simulink model "soc_range_doppler_top"  (R2023b)
settings: Solver=VariableStepAuto  StartTime=0.0  StopTime=stoptime  RelTol=1e-3  EnableMultiTasking=on
PreLoadFcn:
  | soc_range_doppler_init
InitFcn:
  | hsb.blkcb2.defineTypes
  | soc_range_doppler_init
model workspace (MAT data in the model file):
  mmap = soc.memmap.MemoryMap
  mmap.isMapValid = 1
  mmap.controllerInfo = soc.memmap.MemController
  mmap.controllerInfo.memPSRange = {'2', 'G'}
  mmap.controllerInfo.memPLBaseAddr = '0x500000000'
  mmap.controllerInfo.memPLRange = {'4', 'G'}
  mmap.controllerInfo.memPLBaseAddrMMU = {9, '0'}
  mmap.controllerInfo.regBaseAddr = '0xA0000000'
  mmap.controllerInfo.regAddrRange = {'256', 'M'}
  mmap.map(1) = soc.memmap.MapParams
  mmap.map(1).type = 'PS Memory Region'
  mmap.map(1).name = 'AXI4-Stream to Software'
  mmap.map(1).baseAddr = '0x00000000'
  mmap.map(1).range = {'4096', 'K'}
  mmap.map(1).path = 'soc_range_doppler_top/AXI4-Stream to Software'
  mmap.map(2) = soc.memmap.MapParams
  mmap.map(2).type = 'User Component'
  mmap.map(2).name = 'Radar Target Emulator'
  mmap.map(2).baseAddr = '0xA0000000'
  mmap.map(2).range = {'64', 'K'}
  mmap.map(2).path = 'soc_range_doppler_fpga/Radar Target Emulator'
  mmap.map(2).regs(1) = soc.memmap.IPCoreRegParams
  mmap.map(2).regs(1).register = 'HDL Coder registers'
  mmap.map(2).regs(1).offset = '0x0000 - 0x00FF'
  mmap.map(2).regs(1).vectorlength = 'N/A'
  mmap.map(2).regs(1).type = 'Reserved'
  mmap.map(2).regs(1).reserved = 1
  mmap.map(2).regs(2) = soc.memmap.IPCoreRegParams
  mmap.map(2).regs(2).blkname = 'Radar Target Emulator'
  mmap.map(2).regs(2).register = 'Target_Emulator_Doppler_Inc'
  mmap.map(2).regs(2).offset = '0x0100'
  mmap.map(2).regs(2).vectorlength = '4'
  mmap.map(2).regs(2).type = 'Processor write channel'
  mmap.map(2).regs(3) = soc.memmap.IPCoreRegParams
  mmap.map(2).regs(3).blkname = 'Radar Target Emulator'
  mmap.map(2).regs(3).register = 'Target_Emulator_Range_Delay'
  mmap.map(2).regs(3).offset = '0x0120'
  mmap.map(2).regs(3).vectorlength = '4'
  mmap.map(2).regs(3).type = 'Processor write channel'
  mmap.map(2).regs(4) = soc.memmap.IPCoreRegParams
  mmap.map(2).regs(4).blkname = 'Radar Target Emulator'
  mmap.map(2).regs(4).register = 'Target_Emulator_Gain'
  mmap.map(2).regs(4).offset = '0x0140'
  mmap.map(2).regs(4).vectorlength = '4'
  mmap.map(2).regs(4).type = 'Processor write channel'
  mmap.map(2).regs(5) = soc.memmap.IPCoreRegParams
  mmap.map(2).regs(5).blkname = 'Radar Target Emulator'
  mmap.map(2).regs(5).register = 'Target_Emulator_Channel_Enable'
  mmap.map(2).regs(5).offset = '0x0160'
  mmap.map(2).regs(5).vectorlength = '4'
  mmap.map(2).regs(5).type = 'Processor write channel'
  mmap.map(3) = soc.memmap.MapParams
  mmap.map(3).type = 'User Component'
  mmap.map(3).name = 'Range Doppler Tx-Rx'
  mmap.map(3).baseAddr = '0xA0010000'
  mmap.map(3).range = {'64', 'K'}
  mmap.map(3).path = 'soc_range_doppler_fpga/Range Doppler Tx-Rx'
  mmap.map(3).regs(1) = soc.memmap.IPCoreRegParams
  mmap.map(3).regs(1).register = 'HDL Coder registers'
  mmap.map(3).regs(1).offset = '0x0000 - 0x00FF'
  mmap.map(3).regs(1).vectorlength = 'N/A'
  mmap.map(3).regs(1).type = 'Reserved'
  mmap.map(3).regs(1).reserved = 1
  mmap.map(3).regs(2) = soc.memmap.IPCoreRegParams
  mmap.map(3).regs(2).blkname = 'Range Doppler Tx-Rx'
  mmap.map(3).regs(2).register = 'Tx_Gain'
  mmap.map(3).regs(2).offset = '0x0100'
  mmap.map(3).regs(2).vectorlength = '1'
  mmap.map(3).regs(2).type = 'Processor write channel'
  mmap.map(3).regs(3) = soc.memmap.IPCoreRegParams
  mmap.map(3).regs(3).blkname = 'Range Doppler Tx-Rx'
  mmap.map(3).regs(3).register = 'CPI_Start'
  mmap.map(3).regs(3).offset = '0x0104'
  mmap.map(3).regs(3).vectorlength = '1'
  mmap.map(3).regs(3).type = 'Processor write channel'
  mmap.map(3).regs(4) = soc.memmap.IPCoreRegParams
  mmap.map(3).regs(4).blkname = 'Range Doppler Tx-Rx'
  mmap.map(3).regs(4).register = 'CPI_Length'
  mmap.map(3).regs(4).offset = '0x0108'
  mmap.map(3).regs(4).vectorlength = '1'
  mmap.map(3).regs(4).type = 'Processor write channel'
  mmap.map(3).regs(5) = soc.memmap.IPCoreRegParams
  mmap.map(3).regs(5).blkname = 'Range Doppler Tx-Rx'
  mmap.map(3).regs(5).register = 'Rx_Delay_Cycles'
  mmap.map(3).regs(5).offset = '0x010C'
  mmap.map(3).regs(5).vectorlength = '1'
  mmap.map(3).regs(5).type = 'Processor write channel'
  mmap.map(4) = soc.memmap.MapParams
  mmap.map(4).type = 'Implicit Component'
  mmap.map(4).name = 'AXI4-Stream to Software DMA S2MM'
  mmap.map(4).baseAddr = '0xA0020000'
  mmap.map(4).range = {'64', 'K'}
  mmap.map(5) = soc.memmap.MapParams
  mmap.map(5).type = 'Implicit Component'
  mmap.map(5).name = 'RFDataConverter/s_axi'
  mmap.map(5).baseAddr = '0xA3C00000'
  mmap.map(5).range = {'256', 'K'}
  mwTaskManagerKernelLatency = 0
  socicb{1}.Registry = containers.Map
  socicb{1}.Registry.serialization.keys = {34131.0015869}
  socicb{1}.Registry.serialization.values = {1}
  socicb{1}.Registry.serialization.uniformity = 0
  socicb{1}.Registry.serialization.keyType = 'double'
  socicb{1}.Registry.serialization.valueType = 'any'
  socicb{1}.Index = 2
  socicb{2}.Registry = containers.Map
  socicb{2}.Registry.serialization.keys = {}
  socicb{2}.Registry.serialization.values = {}
  socicb{2}.Registry.serialization.uniformity = 0
  socicb{2}.Registry.serialization.keyType = 'double'
  socicb{2}.Registry.serialization.valueType = 'any'
  socicb{2}.Index = 1
  socvcb = containers.Map
  socvcb.serialization.keys = {514.000488281}
  socvcb.serialization.values : function handle (value not decoded)
  socvcb.serialization.uniformity = 0
  socvcb.serialization.keyType = 'double'
  socvcb.serialization.valueType = 'any'
values from neighbouring files (symbols this model uses):
  ConverterSampleRate = 2e9    (= 2000000000)    [soc_range_doppler_init.m]
  FPGAClkRate = Fs/SamplesPerClockCycle    (= 125000000)    [soc_range_doppler_init.m]
  Fs = ConverterSampleRate/DecimInterpFactor    (= 250000000)    [soc_range_doppler_init.m]
  LoopbackDelayCycles = 63    [soc_range_doppler_init.m]
  RxDelayCycles = RngGateSamples/SamplesPerClockCycle + LoopbackDelayCycles*2    [soc_range_doppler_init.m]
  SamplesPerClockCycle = 2    [soc_range_doppler_init.m]
  TsFPGA = 1/FPGAClkRate    (= 8e-09)    [soc_range_doppler_init.m]
  TsHost = 5e-5    (= 5e-05)    [soc_range_doppler_init.m]
  udp_cmd = struct()    [soc_range_doppler_init.m]
undefined symbols (not defined in the file or in its folder): CPILength, D1, D2, I, m, n, P, Q, RngMaxIdx, VelMaxIdx
libraries: prociodatalib x2, dspsrcs4 x2, socmemlib x1, proctasklib x1, xilinxrfsoclib x1
settings Model: ModifiedByFormat=The MathWorks, Inc.  Creator=The MathWorks, Inc.  LastModifiedBy=The MathWorks, Inc.
settings SolverCC: ConcurrentTasks=on  AlgebraicLoopSolver=TrustRegion  PositivePriorityOrder=on  MaxZcPerStep=1
settings DataIOCC: ReturnWorkspaceOutputs=off
settings OptimizationCC: EnhancedBackFolding=on  PassReuseOutputArgsAs=Individual arguments  ZeroExternalMemoryAtStartup=off  ZeroInternalMemoryAtStartup=off  MaxStackSize=64  OptimizeBlockOrder=speed  DifferentSizesBufferReuse=on  OptimizationCustomize=off  EfficientTunableParamExpr=on
settings DebuggingCC: ParameterTunabilityLossMsg=error  UnconnectedInputMsg=warning  UnconnectedOutputMsg=warning  UnconnectedLineMsg=warning
settings HardwareCC: ProdBitPerLong=64  ProdLargestAtomicInteger=LongLong  ProdLargestAtomicFloat=Double  ProdLongLongMode=on  ProdHWDeviceType=ARM Compatible->ARM 64-bit (LP64)  HardwareBoardFeatureSet=SoCBlockset
settings ModelReferenceCC: EnableRefExpFcnMdlSchedulingChecks=on  ModelReferenceNumInstancesAllowed=Single
settings SFSimCC: MATLABDynamicMemAlloc=off
settings RTWCC: Description=Embedded Coder  SystemTargetFile=ert.tlc  HardwareBoard=Xilinx Zynq UltraScale+ RFSoC ZCU111 Evaluation Kit  TLCOptions="-aInlineSetEventsForThisBaseRateFcn=TLC_FALSE -aSuppressMultiTaskScheduler=TLC_FALSE  -aRateBasedStepFcn=0"  TemplateMakefile=ert_default_tmf  Toolchain=Linaro AArch64 Linux v6.3.1  DLArmComputeVersion=19.05
settings CodeAppCC: ForceParamTrailComments=on  IgnoreCustomStorageClasses=off  OperatorAnnotations=on  SimulinkDataObjDesc=on  SFDataObjDesc=on  InsertBlockDesc=on

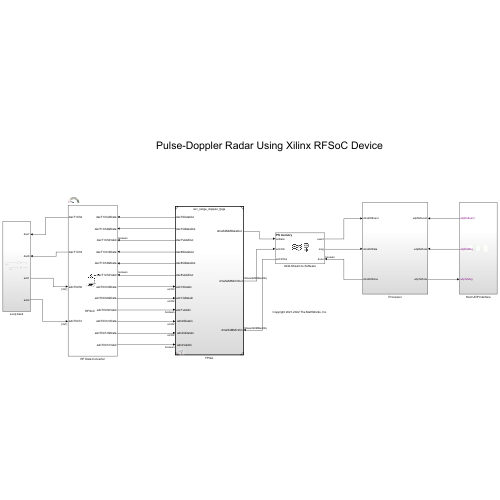
[thumbnail: Simulink's stored preview of the top-level diagram]
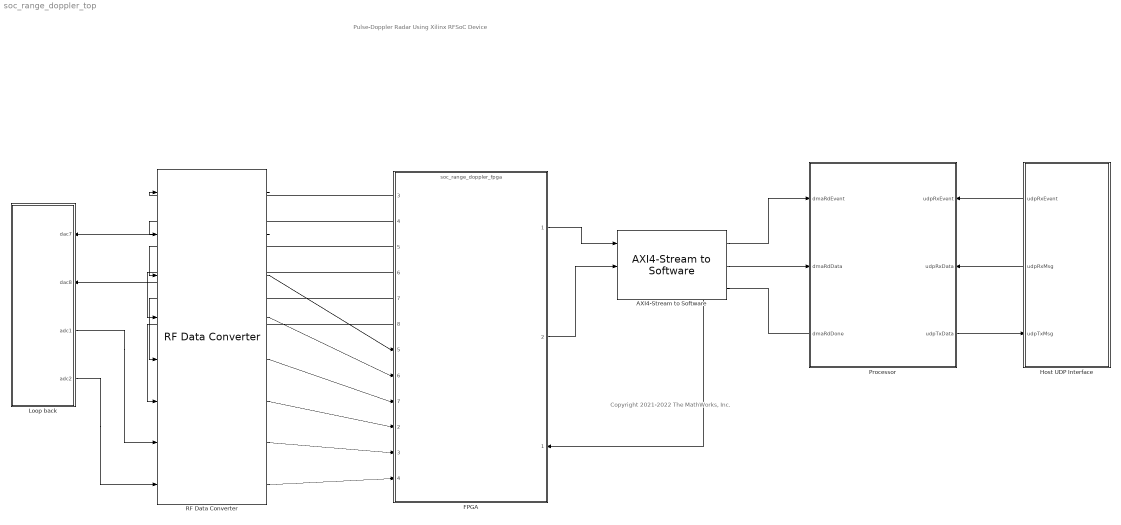
== system soc_range_doppler_top ==
  note: Pulse-Doppler Radar Using Xilinx RFSoC Device
  note: Copyright 2021-2022 The MathWorks, Inc.
  AXI4-Stream to Software : socmemlib/AXI4-Stream to Software  MemorySimulation=Burst accurate  MemorySelection=PS memory  MRNumBuffers=S2MM_DMANumBuffers  BurstLengthWriterChIf=256  FIFODepthWriter=8  FIFOAFullDepthWriter=6  ICClockFrequencyWriter=300  ICDataWidthWriter=64  ChDimensionsWriterChIf=1  ChTypeWriterChIf=uint64  ChFrameSampleTimeWriterChIf=1/FPGAClkRate  ChBitPackedWriterChIf=off  ChDimensionsReaderChIf=S2MM_DMAFrameLength  ChTypeReaderChIf=uint64  LastTargetBoard=Xilinx Zynq UltraScale+ RFSoC ZCU111 Evaluation Kit  MRRegionSize=4194304  MRBufferSize=262144  DiagnosticLevel=No debug
  FPGA : ModelReference  ModelNameDialog=soc_range_doppler_fpga.slx  SimulationMode=Normal  ModelReferenceVersion=1.0
      settings: PortSchema="{\"entries\":[{\"content\":{\"sides\":[{\"content\":{\"connectorIds\":[\"Out3\",\"Out4\",\"Out5\",\"Out6\",\"Out7\",\"Out8\",\"In5\",\"In6\",\"In7\",\"In2\",\"In3\",\"In4\"]},\"type\":\"ConnectorPlacement.EquallySpacedRectSide\",\"uuid\":\"422e8f89-866f-4e63-8b25-cadbd336be37\"},{\"content\":{\"connectorIds\":[\"Out1\",\"Out2\",\"In1\"],\"side\":\"RIGHT\"},\"type\":\"ConnectorPlacement.EquallySpacedRectSide\",\"uuid\":\"dce0ed7e-9928-416e-b2ed-d7d34b81a84a\"},{\"content\":{\"connectorIds\":[],\"side\":\"TOP\"},\"type\":\"ConnectorPlacement.EquallySpacedRectSide\",\"uuid\":\"a6e1b56d-9a0e-41ff-8dbe-5200ba64d569\"}]},\"type\":\"ConnectorPlacement.EquallySpacedConnector\",\"uuid\":\"a650c01e-33da-4d6b-a752-c4fd08663ce5\"}],\"packageUris\":[\"http://schema.mathworks.com/mf0/Connector/R2020b\"],\"version\":\"1.0\"}"
  Host UDP Interface : Subsystem
      settings: PortSchema="{\"entries\":[{\"content\":{\"sides\":[{\"content\":{\"connectorIds\":[\"Out1\",\"Out2\",\"In1\"]},\"type\":\"ConnectorPlacement.EquallySpacedRectSide\",\"uuid\":\"9c3f3ca2-7255-442d-89df-713aeb26e21e\"},{\"content\":{\"connectorIds\":[],\"side\":\"RIGHT\"},\"type\":\"ConnectorPlacement.EquallySpacedRectSide\",\"uuid\":\"e07d2c4c-30b4-495f-acff-78102ba2fb53\"},{\"content\":{\"connectorIds\":[],\"side\":\"TOP\"},\"type\":\"ConnectorPlacement.EquallySpacedRectSide\",\"uuid\":\"853d940a-d21c-462a-929f-98a301461923\"},{\"content\":{\"connectorIds\":[],\"side\":\"HIDDEN\"},\"type\":\"ConnectorPlacement.EquallySpacedRectSide\",\"uuid\":\"ea8c92dd-7626-4add-bd8f-a9d4935d66f8\"}]},\"type\":\"ConnectorPlacement.EquallySpacedConnector\",\"uuid\":\"2455c085-c623-453a-9196-168aa3e9b36f\"}],\"packageUris\":[\"http://schema.mathworks.com/mf0/Connector/R2020b\"],\"version\":\"1.0\"}"
  Loop back : Subsystem
      settings: PortSchema="{\"entries\":[{\"content\":{\"sides\":[{\"content\":{\"connectorIds\":[]},\"type\":\"ConnectorPlacement.EquallySpacedRectSide\",\"uuid\":\"975a5334-a629-4491-b90c-43fa61341479\"},{\"content\":{\"connectorIds\":[\"In1\",\"In2\",\"Out1\",\"Out2\"],\"side\":\"RIGHT\"},\"type\":\"ConnectorPlacement.EquallySpacedRectSide\",\"uuid\":\"05690cce-8672-402a-8253-0f6b9724a041\"},{\"content\":{\"connectorIds\":[],\"side\":\"TOP\"},\"type\":\"ConnectorPlacement.EquallySpacedRectSide\",\"uuid\":\"0d5c0932-fd92-4b6a-b2b9-8137fdfe5c54\"}]},\"type\":\"ConnectorPlacement.EquallySpacedConnector\",\"uuid\":\"05fdaa57-5b6b-4572-a65f-c3b7d5edf9ae\"}],\"packageUris\":[\"http://schema.mathworks.com/mf0/Connector/R2020b\"],\"version\":\"1.0\"}"
  Processor : Subsystem
      settings: PortSchema="{\"entries\":[{\"content\":{\"sides\":[{\"content\":{\"connectorIds\":[\"In1\",\"In2\",\"Out2\"]},\"type\":\"ConnectorPlacement.EquallySpacedRectSide\",\"uuid\":\"fdd8d51e-84cf-4172-ae92-3a2268afb915\"},{\"content\":{\"connectorIds\":[\"In3\",\"In4\",\"Out1\"],\"side\":\"RIGHT\"},\"type\":\"ConnectorPlacement.EquallySpacedRectSide\",\"uuid\":\"e3c7202d-80e2-4cca-8eeb-2f96d776b6b9\"},{\"content\":{\"connectorIds\":[],\"side\":\"TOP\"},\"type\":\"ConnectorPlacement.EquallySpacedRectSide\",\"uuid\":\"d91d78b2-c830-4c1a-8566-0c5cca5f25a7\"}]},\"type\":\"ConnectorPlacement.EquallySpacedConnector\",\"uuid\":\"41410483-7731-4907-8551-24eb7e6a32eb\"}],\"packageUris\":[\"http://schema.mathworks.com/mf0/Connector/R2020b\"],\"version\":\"1.0\"}"
  RF Data Converter : xilinxrfsoclib/RF Data Converter  RFDCSim=Pass-through  tabPromptsCB=0  RFInterface=Customize  digitalInterface=I/Q  dac11Enable=off  dac12Enable=off  dac13Enable=off  dac14Enable=off  dac21Enable=off  dac22Enable=off  dac23Enable=on  dac24Enable=on  dac31Enable=off  dac32Enable=off  dac33Enable=off  dac34Enable=off  dac41Enable=off  dac42Enable=off  dac43Enable=off  dac44Enable=off  matchDACParam=on  dacSampleRate=ConverterSampleRate/1e6  interpolationMode=8  dacSamplesPerCycle=2  dacMixerType=Fine  dacMixerMode=I/Q->Real  dacMixerFrequency=Fs/4  dacNCOFrequency=0.5*ones(1,2)  dacNCOPhase=0*ones(1,2)  invertSyncFilter=off  dacTile1SampleRate=1000  dac11InterpolationMode=2  dac11SamplesPerCycle=2  dac11MixerType=Coarse  dac11MixerMode=I/Q->Real  dac11MixerFrequency=Fs/2  dac11NCOFrequency=0  dac11NCOPhase=0  dac11InvertSyncFilter=off  dac12InterpolationMode=2  dac12SamplesPerCycle=2  dac12MixerType=Coarse  dac12MixerMode=I/Q->Real  dac12MixerFrequency=Fs/2  dac12NCOFrequency=0  dac12NCOPhase=0  dac12InvertSyncFilter=off  dac13InterpolationMode=2  dac13SamplesPerCycle=2  dac13MixerType=Coarse  dac13MixerMode=I/Q->Real  dac13MixerFrequency=Fs/2  dac13NCOFrequency=0  dac13NCOPhase=0  dac13InvertSyncFilter=off  dac14InterpolationMode=2  dac14SamplesPerCycle=2  dac14MixerType=Coarse  dac14MixerMode=I/Q->Real  dac14MixerFrequency=Fs/2  dac14NCOFrequency=0  dac14NCOPhase=0  dac14InvertSyncFilter=off  dacTile2SampleRate=1000  dac21InterpolationMode=2  dac21SamplesPerCycle=2  dac21MixerType=Coarse  dac21MixerMode=I/Q->Real  dac21MixerFrequency=Fs/2  dac21NCOFrequency=0  dac21NCOPhase=0  dac21InvertSyncFilter=off  dac22InterpolationMode=2  dac22SamplesPerCycle=2  dac22MixerType=Coarse  dac22MixerMode=I/Q->Real  dac22MixerFrequency=Fs/2  dac22NCOFrequency=0  dac22NCOPhase=0  dac22InvertSyncFilter=off  dac23InterpolationMode=2  dac23SamplesPerCycle=2  dac23MixerType=Coarse  dac23MixerMode=I/Q->Real  dac23MixerFrequency=Fs/2  dac23NCOFrequency=0  dac23NCOPhase=0  dac23InvertSyncFilter=off  dac24InterpolationMode=2  dac24SamplesPerCycle=2  dac24MixerType=Coarse  dac24MixerMode=I/Q->Real  dac24MixerFrequency=Fs/2  dac24NCOFrequency=0  dac24NCOPhase=0  dac24InvertSyncFilter=off  dacTile3SampleRate=1000  dac31InterpolationMode=2  dac31SamplesPerCycle=2  dac31MixerType=Coarse  dac31MixerMode=I/Q->Real  dac31MixerFrequency=Fs/2  dac31NCOFrequency=0  dac31NCOPhase=0  dac31InvertSyncFilter=off  dac32InterpolationMode=2  dac32SamplesPerCycle=2  dac32MixerType=Coarse  dac32MixerMode=I/Q->Real  dac32MixerFrequency=Fs/2  dac32NCOFrequency=0  dac32NCOPhase=0  dac32InvertSyncFilter=off  dac33InterpolationMode=2  dac33SamplesPerCycle=2  dac33MixerType=Coarse  dac33MixerMode=I/Q->Real  dac33MixerFrequency=Fs/2  dac33NCOFrequency=0  dac33NCOPhase=0  dac33InvertSyncFilter=off  dac34InterpolationMode=2  dac34SamplesPerCycle=2  dac34MixerType=Coarse  dac34MixerMode=I/Q->Real  dac34MixerFrequency=Fs/2  dac34NCOFrequency=0  dac34NCOPhase=0  dac34InvertSyncFilter=off  dacTile4SampleRate=1000  dac41InterpolationMode=2  dac41SamplesPerCycle=2  dac41MixerType=Coarse  dac41MixerMode=I/Q->Real  dac41MixerFrequency=Fs/2  dac41NCOFrequency=0  dac41NCOPhase=0  dac41InvertSyncFilter=off  dac42InterpolationMode=2  dac42SamplesPerCycle=2  dac42MixerType=Coarse  dac42MixerMode=I/Q->Real  dac42MixerFrequency=Fs/2  dac42NCOFrequency=0  dac42NCOPhase=0  dac42InvertSyncFilter=off  dac43InterpolationMode=2  dac43SamplesPerCycle=2  dac43MixerType=Coarse  dac43MixerMode=I/Q->Real  dac43MixerFrequency=Fs/2  dac43NCOFrequency=0  dac43NCOPhase=0  dac43InvertSyncFilter=off  dac44InterpolationMode=2  dac44SamplesPerCycle=2  dac44MixerType=Coarse  dac44MixerMode=I/Q->Real  dac44MixerFrequency=Fs/2  dac44NCOFrequency=0  dac44NCOPhase=0  dac44InvertSyncFilter=off  adc11Enable=on  adc12Enable=on  adc13Enable=off  adc14Enable=off  adc21Enable=off  adc22Enable=off  adc23Enable=off  adc24Enable=off  adc31Enable=off  adc32Enable=off  adc33Enable=off  adc34Enable=off  adc41Enable=off  adc42Enable=off  adc43Enable=off  adc44Enable=off  adcOutUnpackedData=off  matchADCParam=on  adcSampleRate=ConverterSampleRate/1e6  decimationMode=8  adcSamplesPerCycle=2  adcMixerType=Fine  adcMixerMode=Real->I/Q  adcMixerFrequency=-Fs/4  adcNCOFrequency=-0.5*ones(1,2)  adcNCOPhase=0*ones(1,2)  adcTile1SampleRate=1000  adc11DecimationMode=2  adc11SamplesPerCycle=2  adc11MixerType=Coarse  adc11MixerMode=Real->I/Q  adc11MixerFrequency=Fs/2  adc11NCOFrequency=0  adc11NCOPhase=0  adc12DecimationMode=2  adc12SamplesPerCycle=2  adc12MixerType=Coarse  adc12MixerMode=Real->I/Q  adc12MixerFrequency=Fs/2  adc12NCOFrequency=0  adc12NCOPhase=0  adc13DecimationMode=2  adc13SamplesPerCycle=2  adc13MixerType=Coarse  adc13MixerMode=Real->I/Q  adc13MixerFrequency=Fs/2  adc13NCOFrequency=0  adc13NCOPhase=0  adc14DecimationMode=2  adc14SamplesPerCycle=2  adc14MixerType=Coarse  adc14MixerMode=Real->I/Q  adc14MixerFrequency=Fs/2  adc14NCOFrequency=0  adc14NCOPhase=0  adcTile2SampleRate=1000  adc21DecimationMode=2  adc21SamplesPerCycle=2  adc21MixerType=Coarse  adc21MixerMode=Real->I/Q  adc21MixerFrequency=Fs/2  adc21NCOFrequency=0  adc21NCOPhase=0  adc22DecimationMode=2  adc22SamplesPerCycle=2  adc22MixerType=Coarse  adc22MixerMode=Real->I/Q  adc22MixerFrequency=Fs/2  adc22NCOFrequency=0  adc22NCOPhase=0  adc23DecimationMode=2  adc23SamplesPerCycle=2  adc23MixerType=Coarse  adc23MixerMode=Real->I/Q  adc23MixerFrequency=Fs/2  adc23NCOFrequency=0  adc23NCOPhase=0  adc24DecimationMode=2  adc24SamplesPerCycle=2  adc24MixerType=Coarse  adc24MixerMode=Real->I/Q  adc24MixerFrequency=Fs/2  adc24NCOFrequency=0  adc24NCOPhase=0  adcTile3SampleRate=1000  adc31DecimationMode=2  adc31SamplesPerCycle=2  adc31MixerType=Coarse  adc31MixerMode=Real->I/Q  adc31MixerFrequency=Fs/2  adc31NCOFrequency=0  adc31NCOPhase=0  adc32DecimationMode=2  adc32SamplesPerCycle=2  adc32MixerType=Coarse  adc32MixerMode=Real->I/Q  adc32MixerFrequency=Fs/2  adc32NCOFrequency=0  adc32NCOPhase=0  adc33DecimationMode=2  adc33SamplesPerCycle=2  adc33MixerType=Coarse  adc33MixerMode=Real->I/Q  adc33MixerFrequency=Fs/2  adc33NCOFrequency=0  adc33NCOPhase=0  adc34DecimationMode=2  adc34SamplesPerCycle=2  adc34MixerType=Coarse  adc34MixerMode=Real->I/Q  adc34MixerFrequency=Fs/2  adc34NCOFrequency=0  adc34NCOPhase=0  adcTile4SampleRate=1000  adc41DecimationMode=2  adc41SamplesPerCycle=2  adc41MixerType=Coarse  adc41MixerMode=Real->I/Q  adc41MixerFrequency=Fs/2  adc41NCOFrequency=0  adc41NCOPhase=0  adc42DecimationMode=2  adc42SamplesPerCycle=2  adc42MixerType=Coarse  adc42MixerMode=Real->I/Q  adc42MixerFrequency=Fs/2  adc42NCOFrequency=0  adc42NCOPhase=0  adc43DecimationMode=2  adc43SamplesPerCycle=2  adc43MixerType=Coarse  adc43MixerMode=Real->I/Q  adc43MixerFrequency=Fs/2  adc43NCOFrequency=0  adc43NCOPhase=0  adc44DecimationMode=2  adc44SamplesPerCycle=2  adc44MixerType=Coarse  adc44MixerMode=Real->I/Q  adc44MixerFrequency=Fs/2  adc44NCOFrequency=0  adc44NCOPhase=0  multiTileSync=off  externalPLL=off  dacRealTimeNCOPortsEnable=off  adcRealTimeNCOPortsEnable=off  adcRealTimePortsEnable=off  adcThresholdMode=Sticky over  adcThreshold1=0  adcDelayCounter=0  adcThreshold2Mode=Sticky over  adcThreshold2=0  adcThreshold2DelayCounter=0  adc11ThresholdMode=Sticky over  adc11Threshold1=0  adc11DelayCounter=0  adc11Threshold2Mode=Sticky over  adc11Threshold2=0  adc11Threshold2DelayCounter=0  adc12ThresholdMode=Sticky over  adc12Threshold1=0  adc12DelayCounter=0  adc12Threshold2Mode=Sticky over  adc12Threshold2=0  adc12Threshold2DelayCounter=0  adc13ThresholdMode=Sticky over  adc13Threshold1=0  adc13DelayCounter=0  adc13Threshold2Mode=Sticky over  adc13Threshold2=0  adc13Threshold2DelayCounter=0  adc14ThresholdMode=Sticky over  adc14Threshold1=0  adc14DelayCounter=0  adc14Threshold2Mode=Sticky over  adc14Threshold2=0  adc14Threshold2DelayCounter=0  adc21ThresholdMode=Sticky over  adc21Threshold1=0  adc21DelayCounter=0  adc21Threshold2Mode=Sticky over  adc21Threshold2=0  adc21Threshold2DelayCounter=0  adc22ThresholdMode=Sticky over  adc22Threshold1=0  adc22DelayCounter=0  adc22Threshold2Mode=Sticky over  adc22Threshold2=0  adc22Threshold2DelayCounter=0  adc23ThresholdMode=Sticky over  adc23Threshold1=0  adc23DelayCounter=0  adc23Threshold2Mode=Sticky over  adc23Threshold2=0  adc23Threshold2DelayCounter=0  adc24ThresholdMode=Sticky over  adc24Threshold1=0  adc24DelayCounter=0  adc24Threshold2Mode=Sticky over  adc24Threshold2=0  adc24Threshold2DelayCounter=0  adc31ThresholdMode=Sticky over  adc31Threshold1=0  adc31DelayCounter=0  adc31Threshold2Mode=Sticky over  adc31Threshold2=0  adc31Threshold2DelayCounter=0  adc32ThresholdMode=Sticky over  adc32Threshold1=0  adc32DelayCounter=0  adc32Threshold2Mode=Sticky over  adc32Threshold2=0  adc32Threshold2DelayCounter=0  adc33ThresholdMode=Sticky over  adc33Threshold1=0  adc33DelayCounter=0  adc33Threshold2Mode=Sticky over  adc33Threshold2=0  adc33Threshold2DelayCounter=0  adc34ThresholdMode=Sticky over  adc34Threshold1=0  adc34DelayCounter=0  adc34Threshold2Mode=Sticky over  adc34Threshold2=0  adc34Threshold2DelayCounter=0  adc41ThresholdMode=Sticky over  adc41Threshold1=0  adc41DelayCounter=0  adc41Threshold2Mode=Sticky over  adc41Threshold2=0  adc41Threshold2DelayCounter=0  adc42ThresholdMode=Sticky over  adc42Threshold1=0  adc42DelayCounter=0  adc42Threshold2Mode=Sticky over  adc42Threshold2=0  adc42Threshold2DelayCounter=0  adc43ThresholdMode=Sticky over  adc43Threshold1=0  adc43DelayCounter=0  adc43Threshold2Mode=Sticky over  adc43Threshold2=0  adc43Threshold2DelayCounter=0  adc44ThresholdMode=Sticky over  adc44Threshold1=0  adc44DelayCounter=0  adc44Threshold2Mode=Sticky over  adc44Threshold2=0  adc44Threshold2DelayCounter=0
  wires:
  Host UDP Interface/1(udpRxEvent) -> Processor/3(udpRxEvent)
  Processor/1(udpTxData) -> Host UDP Interface/1(udpTxMsg)
  AXI4-Stream to Software/1 -> Processor/1(dmaRdEvent)
  AXI4-Stream to Software/2 -> Processor/2(dmaRdData)
  Host UDP Interface/2(udpRxMsg) -> Processor/4(udpRxData)
  Processor/2(dmaRdDone) -> AXI4-Stream to Software/3
  FPGA/1 -> AXI4-Stream to Software/1
  FPGA/2 -> AXI4-Stream to Software/2
  AXI4-Stream to Software/3 -> FPGA/1
  Loop back/1(adc1) -> RF Data Converter/7
  Loop back/2(adc2) -> RF Data Converter/8
  RF Data Converter/2 -> Loop back/2(dac8)
  RF Data Converter/1 -> Loop back/1(dac7)
  FPGA/3 -> RF Data Converter/1
  FPGA/4 -> RF Data Converter/2
  FPGA/5 -> RF Data Converter/3
  FPGA/6 -> RF Data Converter/4
  FPGA/7 -> RF Data Converter/5
  FPGA/8 -> RF Data Converter/6
  RF Data Converter/3 -> FPGA/5
  RF Data Converter/4 -> FPGA/6
  RF Data Converter/5 -> FPGA/7
  RF Data Converter/6 -> FPGA/2
  RF Data Converter/7 -> FPGA/3
  RF Data Converter/8 -> FPGA/4

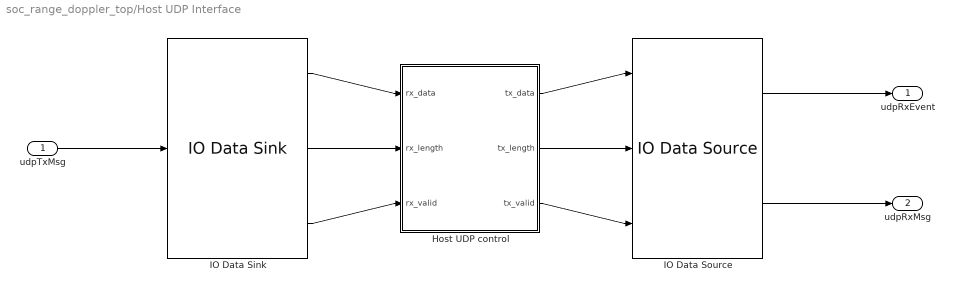
== system soc_range_doppler_top/Host UDP Interface ==
  udpTxMsg : Inport
  Host UDP control : MATLAB Function  TreatAsAtomicUnit=on
  IO Data Sink : prociodatalib/IO Data Sink  OutputSink=To output port  DataTypeStr=single  Dimensions=RngMaxIdx*VelMaxIdx  DeviceType=UDP  EventDataPort=Data  QueueLength=65535  SampleTime=TsHost  EnableDonePort=off
  IO Data Source : prociodatalib/IO Data Source  InputSource=From input port  Value=uint32(1:1024)  ObjectName=[]  DeviceType=UDP  ShowEventPort=off  EventDataPort=Data and Event  QueueLength=1024  DataTypeStr=uint32  Dimensions=1024  ShowDonePort=off  SampleTime=-1  InternalSampleTime=-1
  udpRxEvent : Outport
  udpRxMsg : Outport  Port=2
  wires:
  IO Data Source/2 -> udpRxMsg/1
  IO Data Source/1 -> udpRxEvent/1
  udpTxMsg/1 -> IO Data Sink/1
  IO Data Sink/1 -> Host UDP control/1(rx_data)
  IO Data Sink/2 -> Host UDP control/2(rx_length)
  IO Data Sink/3 -> Host UDP control/3(rx_valid)
  Host UDP control/3(tx_valid) -> IO Data Source/3
  Host UDP control/2(tx_length) -> IO Data Source/2
  Host UDP control/1(tx_data) -> IO Data Source/1

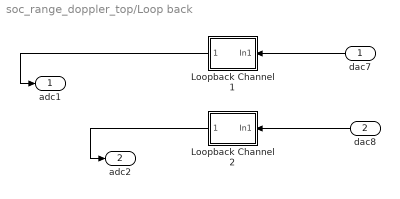
== system soc_range_doppler_top/Loop back ==
  dac7 : Inport
  dac8 : Inport  Port=2
  Loopback Channel 1 : Subsystem
  Loopback Channel 2 : Subsystem
  adc1 : Outport
  adc2 : Outport  Port=2
  wires:
  dac7/1 -> Loopback Channel 1/1(In1)
  Loopback Channel 2/1(Out1) -> adc2/1
  dac8/1 -> Loopback Channel 2/1(In1)
  Loopback Channel 1/1(Out1) -> adc1/1

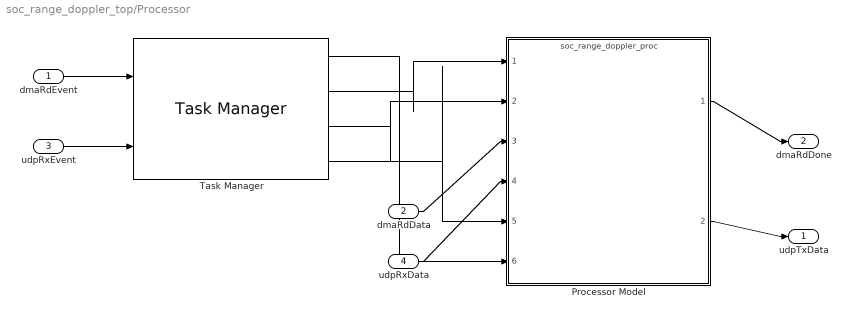
== system soc_range_doppler_top/Processor ==
  dmaRdEvent : Inport
  dmaRdData : Inport  Port=2
  udpRxEvent : Inport  Port=3
  udpRxData : Inport  Port=4
  Processor Model : ModelReference  InputPortMessageModes=n,n,m,m,n,n  OutputPortMessageModes=m,m  ModelNameDialog=soc_range_doppler_proc.slx  SimulationMode=Normal  ScheduleRates=on  CachedPortDiscreteRates=[0.01;0.2]  ModelEventPortInfo=P:D1[0.01][0][0],P:D2[0.2][0][0]  ModelReferenceVersion=1.0
  Task Manager : proctasklib/Task Manager  AllTaskData="[{\"taskName\":\"baseRateTask\",\"taskType\":\"Timer-driven\",\"taskEvent\":\"baseRateTaskEvent\",\"taskPeriod\":\"TsSWBase\",\"taskPriority\":\"51\",\"coreSelection\":\"Specified core\",\"coreNum\":\"0\",\"dropOverranTasks\":false,\"playbackRecorded\":false,\"diagnosticsFile\":\"\",\"taskDurationSource\":\"Dialog\",\"taskDuration\":1E-6,\"taskDurationDeviation\":0,\"logExecutionData\":true,\"logDroppedTasks\":false,\"version\":\"2.6\",\"taskDurationData\":{\"percent\":\"100\",\"mean\":\"1e-06\",\"dev\":\"0\",\"min\":\"1e-06\",\"max\":\"1e-06\"},\"taskEventSource\":\"Internal\",\"taskEventSourceAssignmentType\":\"AutoAssigned\",\"taskEventSourceType\":\"Unspecified\",\"taskEventGroup\":\"Unspecified\",\"taskEventInterrupt\":\"Unspecified\",\"taskEventOrder\":1,\"taskDisablePremption\":false,\"taskClearInterruptFlagsAtEndOfEvent\":false},{\"taskName\":\"dataReadTask\",\"taskType\":\"Event-driven\",\"taskEvent\":\"dataReadTaskEvent\",\"taskPeriod\":\"0.1\",\"taskPriority\":\"50\",\"coreSelection\":\"Specified core\",\"coreNum\":\"1\",\"dropOverranTasks\":false,\"playbackRecorded\":false,\"diagnosticsFile\":\"\",\"taskDurationSource\":\"Dialog\",\"taskDuration\":1E-6,\"taskDurationDeviation\":0,\"logExecutionData\":true,\"logDroppedTasks\":false,\"version\":\"2.6\",\"taskDurationData\":{\"percent\":[\"100\"],\"mean\":[\"10e-6\"],\"dev\":[\"0\"],\"min\":[\"8e-6\"],\"max\":[\"12e-6\"]},\"taskEventSource\":\"AXI4-Stream to Software\",\"taskEventSourceAssignmentType\":\"AutoAssigned\",\"taskEventSourceType\":\"Stream\",\"taskEventGroup\":\"Unspecified\",\"taskEventInterrupt\":\"Unspecified\",\"taskEventOrder\":1,\"taskDisablePremption\":false,\"taskClearInterruptFlagsAtEndOfEvent\":false},{\"taskName\":\"udpRxTask\",\"taskType\":\"Event-driven\",\"taskEvent\":\"udpRxTaskEvent\",\"taskPeriod\":\"0.1\",\"taskPriority\":\"45\",\"coreSelection\":\"Specified core\",\"coreNum\":\"0\",\"dropOverranTasks\":false,\"playbackRecorded\":false,\"diagnosticsFile\":\"\",\"taskDurationSource\":\"Dialog\",\"taskDuration\":1E-6,\"taskDurationDeviation\":0,\"logExecutionData\":true,\"logDroppedTasks\":false,\"version\":\"2.6\",\"taskDurationData\":{\"percent\":[\"100\"],\"mean\":[\"1.55e-6\"],\"dev\":[\"0\"],\"min\":[\"1.5e-6\"],\"max\":[\"1.6e-6\"]},\"taskEventSource\":\"IO Data Source\",\"taskEventSourceAssignmentType\":\"AutoAssigned\",\"taskEventSourceType\":\"\",\"taskEventGroup\":\"Unspecified\",\"taskEventInterrupt\":\"Unspecified\",\"taskEventOrder\":1,\"taskDisablePremption\":false,\"taskClearInterruptFlagsAtEndOfEvent\":false},{\"taskName\":\"radarTargetUpdateTask\",\"taskType\":\"Timer-driven\",\"taskEvent\":\"newTask1Event\",\"taskPeriod\":\"TsTargetUpdate\",\"taskPriority\":\"51\",\"coreSelection\":\"Specified core\",\"coreNum\":\"2\",\"dropOverranTasks\":false,\"playbackRecorded\":false,\"diagnosticsFile\":\"\",\"taskDurationSource\":\"Dialog\",\"taskDuration\":1E-6,\"taskDurationDeviation\":0,\"logExecutionData\":true,\"logDroppedTasks\":false,\"version\":\"2.6\",\"taskDurationData\":{\"percent\":\"100\",\"mean\":\"1e-06\",\"dev\":\"0\",\"min\":\"1e-06\",\"max\":\"1e-06\"},\"taskEventSource\":\"Internal\",\"taskEventSourceAssignmentType\":\"AutoAssigned\",\"taskEventSourceType\":\"Unspecified\",\"taskEventGroup\":\"Unspecified\",\"taskEventInterrupt\":\"Unspecified\",\"taskEventOrder\":1,\"taskDisablePremption\":false,\"taskClearInterruptFlagsAtEndOfEvent\":false}]"  EnableTaskSimulation=on  StreamToSDI=on  WriteToFile=off  OverwriteFile=off  SupportEventPorts=on  UseScheduleEditor=off  CustomizationInfo=''
  udpTxData : Outport
  dmaRdDone : Outport  Port=2
  wires:
  Processor Model/1 -> dmaRdDone/1
  dmaRdData/1 -> Processor Model/3
  udpRxData/1 -> Processor Model/4
  Processor Model/2 -> udpTxData/1
  dmaRdEvent/1 -> Task Manager/1
  udpRxEvent/1 -> Task Manager/2
  Task Manager/2 -> Processor Model/1
  Task Manager/3 -> Processor Model/2
  Task Manager/1 -> Processor Model/6
  Task Manager/4 -> Processor Model/5

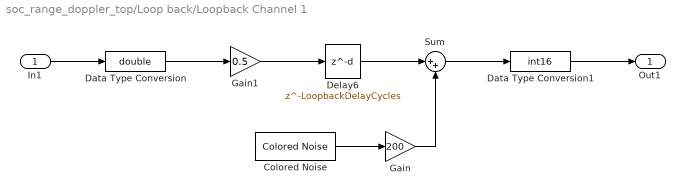
== system soc_range_doppler_top/Loop back/Loopback Channel 1 ==
  In1 : Inport
  Colored Noise : dspsrcs4/Colored Noise  Color=white  InverseFrequencyPower=1  BoundedOutput=off  NumChannels=1  OutputDataType=double  SamplesPerFrame=SamplesPerClockCycle*2  SampleTime=TsFPGA/(SamplesPerClockCycle*2)  RandomStream=mt19937ar with seed  Seed=68  SimulateUsing=Interpreted execution
  Data Type Conversion : DataTypeConversion  OutDataTypeStr=double  SaturateOnIntegerOverflow=off  RndMeth=Floor
  Data Type Conversion1 : DataTypeConversion  OutDataTypeStr=int16  SaturateOnIntegerOverflow=off  RndMeth=Floor
  Delay6 : Delay  DelayLength=LoopbackDelayCycles
  Gain : Gain  Gain=200
  Gain1 : Gain  Gain=0.5
  Sum : Sum  Inputs=|++
  Out1 : Outport
  wires:
  Gain1/1 -> Delay6/1
  In1/1 -> Data Type Conversion/1
  Data Type Conversion/1 -> Gain1/1
  Data Type Conversion1/1 -> Out1/1
  Delay6/1 -> Sum/1
  Colored Noise/1 -> Gain/1
  Gain/1 -> Sum/2
  Sum/1 -> Data Type Conversion1/1

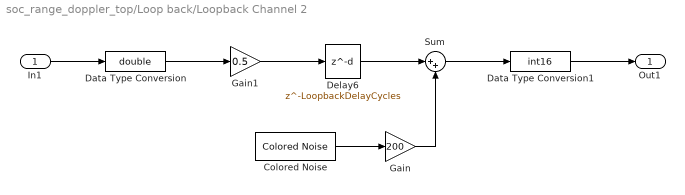
== system soc_range_doppler_top/Loop back/Loopback Channel 2 ==
  In1 : Inport
  Colored Noise : dspsrcs4/Colored Noise  Color=white  InverseFrequencyPower=1  BoundedOutput=off  NumChannels=1  OutputDataType=double  SamplesPerFrame=SamplesPerClockCycle*2  SampleTime=TsFPGA/(SamplesPerClockCycle*2)  RandomStream=mt19937ar with seed  Seed=67  SimulateUsing=Interpreted execution
  Data Type Conversion : DataTypeConversion  OutDataTypeStr=double  SaturateOnIntegerOverflow=off  RndMeth=Floor
  Data Type Conversion1 : DataTypeConversion  OutDataTypeStr=int16  SaturateOnIntegerOverflow=off  RndMeth=Floor
  Delay6 : Delay  DelayLength=LoopbackDelayCycles
  Gain : Gain  Gain=200
  Gain1 : Gain  Gain=0.5
  Sum : Sum  Inputs=|++
  Out1 : Outport
  wires:
  Sum/1 -> Data Type Conversion1/1
  Gain/1 -> Sum/2
  Colored Noise/1 -> Gain/1
  Delay6/1 -> Sum/1
  Data Type Conversion1/1 -> Out1/1
  Data Type Conversion/1 -> Gain1/1
  In1/1 -> Data Type Conversion/1
  Gain1/1 -> Delay6/1

== matlab function soc_range_doppler_top/Host UDP Interface/Host UDP control ==
  data: rx_data input; rx_length input; rx_valid input; tx_data output; tx_length output; tx_valid output; udp_cmd parameter; RxDelayCycles parameter; CPILength parameter; VelMaxIdx parameter; RngMaxIdx parameter
function [tx_data,tx_length,tx_valid] = ...
    udp_host(rx_data,rx_length,rx_valid,...
    udp_cmd,RxDelayCycles,CPILength,VelMaxIdx,RngMaxIdx)

coder.extrinsic('hostInitDisplay','hostDetectTargets','displayRangeDoppler');

persistent init_stage hDisp
if isempty(init_stage)
    init_stage = int32(0);
    hDisp = hostInitDisplay;
end

tx_data = zeros(1,udp_cmd.MessageLength);
tx_length = 2;
tx_valid = false;

% Initialization stage
if init_stage < 5
    switch init_stage
        case 0
            tx_data(1:2) = [udp_cmd.Rx_Delay_Cycles RxDelayCycles];
        case 1
            tx_data(1:2) = [udp_cmd.Tx_Gain 1];
        case 2
            tx_data(1:2) = [udp_cmd.CPI_Length CPILength];
        case 3
            tx_data(1:2) = [udp_cmd.CPI_Start 1];
        case 4
            tx_data(1:2) = [udp_cmd.CPI_Start 0];
    end
    tx_valid = true;
    init_stage = init_stage+1;
else
% Active stage
    if rx_valid && (rx_length == RngMaxIdx*VelMaxIdx)
        tx_data(1:2) = [udp_cmd.CPI_Start 1];
        tx_valid = true;
        RngDopplerMap = fftshift(reshape(rx_data,[VelMaxIdx RngMaxIdx]).',2);
        DetectionIdx = hostDetectTargets(RngDopplerMap);
        displayRangeDoppler(RngDopplerMap,DetectionIdx,hDisp);
    end
end
